simulink model "BalancingRobot"  (R2020a)
settings: Solver=FixedStepAuto  StartTime=0.0  StopTime=inf  FixedStep=.001  RelTol=1e-3  EnableMultiTasking=on
libraries: GPIO_Lib x9, REG_Lib x6, simulink x3, TIMERS_Lib x3, USART_Lib x1, STM32_Config_Lib x1
settings Model: Creator=brunj  LastModifiedBy=tuziz
settings DataIOCC: LimitDataPoints=on  SaveFormat=Array  ReturnWorkspaceOutputs=off
settings OptimizationCC: DefaultParameterBehavior=Inlined  PassReuseOutputArgsAs=Individual arguments  LifeSpan=1  EfficientTunableParamExpr=on
settings DebuggingCC: UnderspecifiedInitializationDetection=Classic  MergeDetectMultiDrivingBlocksExec=none  SolverPrmCheckMsg=warning  AllowSymbolicDim=off  StrictBusMsg=ErrorOnBusTreatedAsVector  SFUnexpectedBacktrackingDiag=warning  SFNoUnconditionalDefaultTransitionDiag=warning  SFUndirectedBroadcastEventsDiag=error  SFExecutionAtInitializationDiag=none  ArithmeticOperatorsInVariantConditions=warning
settings HardwareCC: ProdBitPerPointer=32  ProdBitPerSizeT=32  ProdBitPerPtrDiffT=32  ProdLargestAtomicInteger=Integer  ProdWordSize=32  ProdHWDeviceType=STMicroelectronics->STM32 32-bit Cortex-M
settings ModelReferenceCC: PropagateSignalLabelsOutOfModel=off
settings SFSimCC: SimUseLocalCustomCode=off  CompileTimeRecursionLimit=0  EnableRuntimeRecursion=off  MATLABDynamicMemAlloc=off  CustomCodeUndefinedFunction=UseInterfaceOnly
settings RTWCC: Description=stm32 (Embedded Target)  SystemTargetFile=stm32.tlc  TemplateMakefile=stm32.tmf  RTWUseLocalCustomCode=off  IncludeHyperlinkInReport=on
settings CodeAppCC: IgnoreCustomStorageClasses=off  CustomSymbolStrType=$N$R$M  SimulinkBlockComments=off
settings STFCustomTargetCC: ParMdlRefBuildCompliant=on  IncludeMdlTerminateFcn=off  CombineOutputUpdateFcns=on  ERTCustomFileBanners=on  SupportNonFinite=off  SupportComplex=off  SupportContinuousTime=off  SupportNonInlinedSFcns=off  RemoveResetFunc=on  ParenthesesLevel=Maximum  CastingMode=Standards  MATLABClassNameForMDSCustomization=Simulink.SoftwareTarget.ERTCustomization  SystemTargetFile=stm32.tlc
settings ERTTargetCC: MultiwordLength=2048  CompOptLevelCompliant=off  ConcurrentExecutionCompliant=off  IncludeMdlTerminateFcn=off  SupportNonFinite=off  SupportComplex=off  ParenthesesLevel=Maximum  CastingMode=Standards  ModelStepFunctionPrototypeControlCompliant=off  CPPClassGenCompliant=off  UseToolchainInfoCompliant=off  ExtModeTransport=1  ExtModeStaticAllocSize=256  ExtModeMexArgs=0,1,115200,10  InlinedParameterPlacement=NonHierarchical  ERTSrcFileBannerTemplate=sourceFileTemplate.cgt  ERTHdrFileBannerTemplate=sourceFileTemplate.cgt  ERTDataSrcFileTemplate=sourceFileTemplate.cgt  ERTDataHdrFileTemplate=sourceFileTemplate.cgt  ERTCustomFileTemplate=customRoutineProcess.tlc  ConvertIfToSwitch=off  SuppressUnreachableDefaultCases=off  EnableSignedLeftShifts=off  EnableSignedRightShifts=off
settings ConfigComp: CovMetricSettings=dw  CovHtmlReporting=on  CovSaveCumulativeToWorkspaceVar=on  CovSaveSingleToWorkspaceVar=on  CovExternalEMLEnable=off  CovSFcnEnable=off

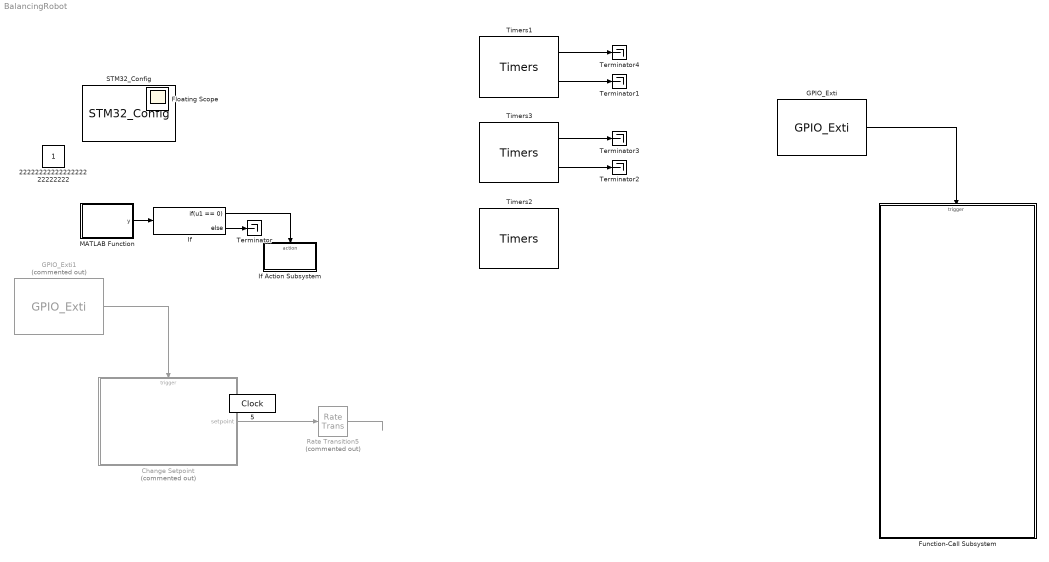
== system BalancingRobot ==
  Change Setpoint : Subsystem  Commented=on  TreatAsAtomicUnit=on
  Function-Call Subsystem : Subsystem  TreatAsAtomicUnit=on
  GPIO_Exti : GPIO_Lib/GPIO_Exti  Port_name=GPIOE  Pin_0=off  Pin_1=on  Pin_2=off  Pin_3=off  Pin_4=off  Pin_5=off  Pin_6=off  Pin_7=off  Pin_8=off  Pin_9=off  Pin_10=off  Pin_11=off  Pin_12=off  Pin_13=off  Pin_14=off  Pin_15=off  PinList=GPIOA0GPIOE1
      settings: SourceProductName=Target Support Package - STM32 Adapter
  GPIO_Exti1 : GPIO_Lib/GPIO_Exti  Commented=on  Port_name=GPIOA  Pin_0=on  Pin_1=off  Pin_2=off  Pin_3=off  Pin_4=off  Pin_5=off  Pin_6=off  Pin_7=off  Pin_8=off  Pin_9=off  Pin_10=off  Pin_11=off  Pin_12=off  Pin_13=off  Pin_14=off  Pin_15=off  PinList=GPIOA0GPIOE1
      settings: SourceProductName=Target Support Package - STM32 Adapter
  If : If  IfExpression=u1 == 0
  If Action Subsystem : Subsystem  TreatAsAtomicUnit=on
  MATLAB Function : MATLAB Function  TreatAsAtomicUnit=on
  Rate Transition5 : RateTransition  Commented=on  Deterministic=off
  STM32_Config : STM32_Config_Lib/STM32_Config  Priority=0  Project_Path=.\  Config_File=BalancingRobot.ioc  MCU_Name=STM32F407VGTx
      settings: SourceProductName=Target Support Package - STM32 Adapter
  Terminator{,1..4} (5 alike) : Terminator
  Timers1 : TIMERS_Lib/Timers  currentTIM=TIM3  TIM_Name=TIM3  sysUsingTimer=off  TIM_APBClock=84000000  TIM_Set_Clk=off  TIM_Prescaler=840-1  TIM_Clock=100000.00  Variable_frequency=off  TIM_Set_OutFreq=off  TIM_ARR=2000  Output_frequency=50.00  Repetition_counter=0  TIM_Mode=Up  TIM_DMA=none  TIM_IRQ=off  TIM_IRQ_ONLY=off  TIM_UP=off  TIM_TRG=off  TIM_COM=off  TIM_BRK=off  NbTIM=3  CH1_enable=on  CH1N_enable=off  CH1_type=Input_Capture  CH1_DMA=off  CH1_int=on  CH1_edge=Rising  CH1_div=1  CH1_variable_duty=off  CH1_set_pulse=off  CH1_output_duty=0.00  CH1_pulse=0  CH2_enable=off  CH2N_enable=off  CH2_type=Input_Capture  CH2_DMA=off  CH2_int=off  CH2_edge=Rising  CH2_div=1  CH2_variable_duty=off  CH2_set_pulse=off  CH2_output_duty=0.00  CH2_pulse=0  CH3_enable=off  CH3N_enable=off  CH3_type=Unknown  CH3_DMA=off  CH3_int=off  CH3_edge=Rising  CH3_div=1  CH3_variable_duty=off  CH3_set_pulse=off  CH3_output_duty=0.00  CH3_pulse=0  CH4_enable=off  CH4N_enable=off  CH4_type=Unknown  CH4_DMA=off  CH4_int=off  CH4_edge=Rising  CH4_div=1  CH4_variable_duty=off  CH4_set_pulse=off  CH4_output_duty=0.00  CH4_pulse=0
      settings: SourceProductName=Target Support Package - STM32 Adapter
  Timers2 : TIMERS_Lib/Timers  currentTIM=TIM9  TIM_Name=TIM9  sysUsingTimer=off  TIM_APBClock=168000000  TIM_Set_Clk=off  TIM_Prescaler=3359  TIM_Clock=50000.00  Variable_frequency=off  TIM_Set_OutFreq=off  TIM_ARR=100  Output_frequency=500.00  Repetition_counter=0  TIM_Mode=Up  TIM_DMA=none  TIM_IRQ=off  TIM_IRQ_ONLY=off  TIM_UP=off  TIM_TRG=off  TIM_COM=off  TIM_BRK=off  NbTIM=3  CH1_enable=on  CH1N_enable=off  CH1_type=Output_PWM  CH1_DMA=off  CH1_int=off  CH1_edge=Rising  CH1_div=1  CH1_variable_duty=off  CH1_set_pulse=off  CH1_output_duty=0.00  CH1_pulse=0  CH2_enable=on  CH2N_enable=off  CH2_type=Output_PWM  CH2_DMA=off  CH2_int=off  CH2_edge=Rising  CH2_div=1  CH2_variable_duty=off  CH2_set_pulse=off  CH2_output_duty=0.00  CH2_pulse=0  CH3_enable=off  CH3N_enable=off  CH3_type=Unknown  CH3_DMA=off  CH3_int=off  CH3_edge=Rising  CH3_div=1  CH3_variable_duty=off  CH3_set_pulse=off  CH3_output_duty=0.00  CH3_pulse=0  CH4_enable=off  CH4N_enable=off  CH4_type=Unknown  CH4_DMA=off  CH4_int=off  CH4_edge=Rising  CH4_div=1  CH4_variable_duty=off  CH4_set_pulse=off  CH4_output_duty=0.00  CH4_pulse=0
      settings: SourceProductName=Target Support Package - STM32 Adapter
  Timers3 : TIMERS_Lib/Timers  currentTIM=TIM2  TIM_Name=TIM2  sysUsingTimer=off  TIM_APBClock=84000000  TIM_Set_Clk=off  TIM_Prescaler=840-1  TIM_Clock=100000.00  Variable_frequency=off  TIM_Set_OutFreq=off  TIM_ARR=2000  Output_frequency=50.00  Repetition_counter=0  TIM_Mode=Up  TIM_DMA=none  TIM_IRQ=off  TIM_IRQ_ONLY=off  TIM_UP=off  TIM_TRG=off  TIM_COM=off  TIM_BRK=off  NbTIM=3  CH1_enable=on  CH1N_enable=off  CH1_type=Input_Capture  CH1_DMA=off  CH1_int=on  CH1_edge=Rising  CH1_div=1  CH1_variable_duty=off  CH1_set_pulse=off  CH1_output_duty=0.00  CH1_pulse=0  CH2_enable=off  CH2N_enable=off  CH2_type=Unknown  CH2_DMA=off  CH2_int=off  CH2_edge=Rising  CH2_div=1  CH2_variable_duty=off  CH2_set_pulse=off  CH2_output_duty=0.00  CH2_pulse=0  CH3_enable=off  CH3N_enable=off  CH3_type=Unknown  CH3_DMA=off  CH3_int=off  CH3_edge=Rising  CH3_div=1  CH3_variable_duty=off  CH3_set_pulse=off  CH3_output_duty=0.00  CH3_pulse=0  CH4_enable=off  CH4N_enable=off  CH4_type=Unknown  CH4_DMA=off  CH4_int=off  CH4_edge=Rising  CH4_div=1  CH4_variable_duty=off  CH4_set_pulse=off  CH4_output_duty=0.00  CH4_pulse=0
      settings: SourceProductName=Target Support Package - STM32 Adapter
  2222222222222222222222222 : Constant  IOType=siggen
  5 : DigitalClock  IOType=siggen
  Floating Scope : Scope
  wires:
  MATLAB Function/1(y) -> If/1
  If/1 -> If Action Subsystem/Action
  If/2 -> Terminator/1
  GPIO_Exti/1 -> Function-Call Subsystem/Trigger
  Rate Transition5/1 -> ?
  Change Setpoint/1(setpoint) -> Rate Transition5/1
  Timers1/1 -> Terminator4/1
  Timers3/2 -> Terminator2/1
  Timers3/1 -> Terminator3/1
  GPIO_Exti1/1 -> Change Setpoint/Trigger
  Timers1/2 -> Terminator1/1

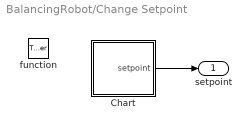
== system BalancingRobot/Change Setpoint ==
  function : TriggerPort  TriggerType=function-call  VariantControl=Variant  OutputDataType=int8
  Chart : Stateflow chart  TreatAsAtomicUnit=on
  setpoint : Outport
  wires:
  Chart/1(setpoint) -> setpoint/1

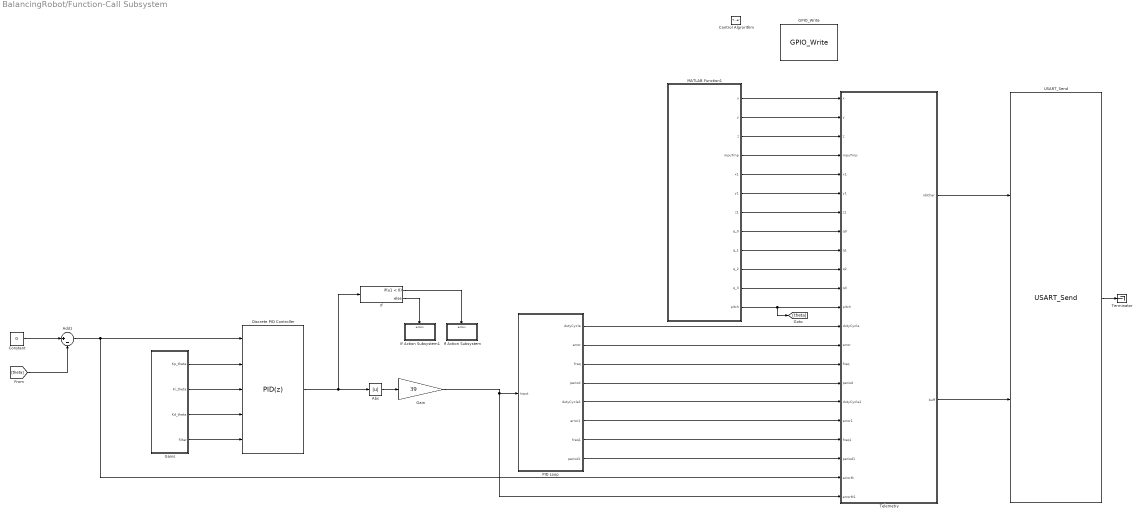
== system BalancingRobot/Function-Call Subsystem ==
  Control Algrorithm : TriggerPort  TriggerType=function-call  VariantControl=Variant
  Abs : Abs
  Add1 : Sum  Inputs=|+-  OutDataTypeStr=double
  Constant : Constant  Value=0
  Discrete PID Controller : simulink/Continuous/PID Controller  Controller=PID  Form=Parallel  TimeDomain=Discrete-time  UseExternalTs=off  SampleTime=-1  IntegratorMethod=Forward Euler  FilterMethod=Forward Euler  ControllerParametersSource=external  P=50.0  I=5  D=.5  UseFilter=on  N=100  TunerSelectOption=Transfer Function Based (PID Tuner App)  InitialConditionSource=internal  InitialConditionForIntegrator=0  InitialConditionForFilter=0  DifferentiatorICPrevScaledInput=0  ExternalReset=none  TrackingMode=off  Kt=1  LimitOutput=on  UpperSaturationLimit=39  LowerSaturationLimit=-39  LinearizeAsGain=off  AntiWindupMode=clamping  Kb=1  POutMin=[]  POutMax=[]  IOutMin=[]  IOutMax=[]  DOutMin=[]  DOutMax=[]  NOutMin=[]  NOutMax=[]  SumOutMin=[]  SumOutMax=[]  SaturationOutMin=[]  SaturationOutMax=[]  PParamMin=[]  PParamMax=[]  IParamMin=[]  IParamMax=[]  DParamMin=[]  DParamMax=[]  NParamMin=[]  NParamMax=[]  KbParamMin=[]  KbParamMax=[]  KtParamMin=[]  KtParamMax=[]  KbOutMin=[]  KbOutMax=[]  KtOutMin=[]  KtOutMax=[]  IntegratorOutMin=[]  IntegratorOutMax=[]  FilterOutMin=[]  FilterOutMax=[]  SumI1OutMin=[]  SumI1OutMax=[]  SumI2OutMin=[]  SumI2OutMax=[]  SumI3OutMin=[]  SumI3OutMax=[]  SumI4OutMin=[]  SumI4OutMax=[]  SumDOutMin=[]  SumDOutMax=[]  DifferentiatorOutMin=[]  DifferentiatorOutMax=[]  FilterDiffOutCoefMin=[]  FilterDiffOutCoefMax=[]  ReciprocalOutMin=[]  ReciprocalOutMax=[]  SumDenOutMin=[]  SumDenOutMax=[]  SumNumOutMin=[]  SumNumOutMax=[]  DivideOutMin=[]  DivideOutMax=[]  UdiffTsProdOutMin=[]  UdiffTsProdOutMax=[]  NTsProdOutMin=[]  NTsProdOutMax=[]  UintegralTsProdOutMin=[]  UintegralTsProdOutMax=[]  UngainTsProdOutMin=[]  UngainTsProdOutMax=[]  IntegratorContinuousStateAttributes=''  IntegratorStateMustResolveToSignalObject=off  IntegratorRTWStateStorageClass=Auto  FilterContinuousStateAttributes=''  FilterStateMustResolveToSignalObject=off  FilterRTWStateStorageClass=Auto  ParallelPVariant=ExternalParameters  IdealPVariant=Disabled  IVariant=ExternalParameters  DVariant=ExternalParameters  IntegratorVariant=Discrete  SatVariant=Enabled  AWVariant=DiscClampingParallel  PCopyVariant=Disabled  TRVariant=Disabled  FdbkBlocksVariant=Forward  IdealPFdbkVariant=Disabled  SatFdbkVariant=Disabled  DerivativeFilterVariant=ForwardEulerFilter  NVariant=ExternalParameters  NCopyVariant=Disabled  FilterICVariant=InternalICsFilter  IntegratorICVariant=InternalICs  ExternalResetVariant=Disabled  TRSumVariant=Passthrough  SumFdbkVariant=Disabled  SumVariant=Sum_PID  TsampFilterVariant=InternalTs  TsampNgainVariant=Passthrough  TsampIntegralVariant=Passthrough
  GPIO_Write : GPIO_Lib/GPIO_Write  Port_name=GPIOD  Pin0=off  Toggle_Pin0=off  Pin1=off  Toggle_Pin1=off  Pin2=off  Toggle_Pin2=off  Pin3=off  Toggle_Pin3=off  Pin4=off  Toggle_Pin4=off  Pin5=off  Toggle_Pin5=off  Pin6=off  Toggle_Pin6=off  Pin7=off  Toggle_Pin7=off  Pin8=off  Toggle_Pin8=off  Pin9=off  Toggle_Pin9=off  Pin10=off  Toggle_Pin10=off  Pin11=off  Toggle_Pin11=off  Pin12=off  Toggle_Pin12=off  Pin13=off  Toggle_Pin13=off  Pin14=off  Toggle_Pin14=off  Pin15=on  Toggle_Pin15=on  PinList="GPIOD1   2   3   4  12  13  14  15"
      settings: SourceProductName=Target Support Package - STM32 Adapter
  Gain : Gain  Gain=39
  Gains : MATLAB Function  TreatAsAtomicUnit=on
  If : If  IfExpression=u1 < 0
  If Action Subsystem : Subsystem  TreatAsAtomicUnit=on
  If Action Subsystem1 : Subsystem  TreatAsAtomicUnit=on
  MATLAB Function1 : MATLAB Function  Priority=0  TreatAsAtomicUnit=on
  PID Loop : Subsystem  TreatAsAtomicUnit=on
  Telemetry : MATLAB Function  TreatAsAtomicUnit=on
  Terminator : Terminator
  USART_Send : USART_Lib/USART_Send  USART_name=USART3  Buff_size=199  nbUsart=1  usartMode=Asynchronous  usartDma_Rx=off  usartDma_Tx=off  usartIt=on
      settings: SourceProductName=Target Support Package - STM32 Adapter
  wires:
  Telemetry/2(buff) -> USART_Send/2
  Telemetry/1(nbChar) -> USART_Send/1
  USART_Send/1 -> Terminator/1
  MATLAB Function1/3(z) -> Telemetry/3(z)
  MATLAB Function1/1(x) -> Telemetry/1(x)
  MATLAB Function1/2(y) -> Telemetry/2(y)
  MATLAB Function1/4(mpuTmp) -> Telemetry/4(mpuTmp)
  MATLAB Function1/5(x1) -> Telemetry/5(x1)
  MATLAB Function1/6(y1) -> Telemetry/6(y1)
  MATLAB Function1/7(z1) -> Telemetry/7(z1)
  MATLAB Function1/8(q_0) -> Telemetry/8(q0)
  MATLAB Function1/9(q_1) -> Telemetry/9(q1)
  MATLAB Function1/10(q_2) -> Telemetry/10(q2)
  MATLAB Function1/11(q_3) -> Telemetry/11(q3)
  MATLAB Function1/12(pitch) -> [theta], Telemetry/12(pitch)
  PID Loop/1(dutyCycle) -> Telemetry/13(dutyCycle)
  PID Loop/2(error) -> Telemetry/14(error)
  PID Loop/3(freq) -> Telemetry/15(freq)
  PID Loop/4(period) -> Telemetry/16(period)
  PID Loop/5(dutyCycle1) -> Telemetry/17(dutyCycle1)
  PID Loop/6(error1) -> Telemetry/18(error1)
  PID Loop/7(freq1) -> Telemetry/19(freq1)
  PID Loop/8(period1) -> Telemetry/20(period1)
  If/1 -> If Action Subsystem/Action
  If/2 -> If Action Subsystem1/Action
  Discrete PID Controller/1 -> If/1, Abs/1
  Add1/1 -> Discrete PID Controller/1, Telemetry/21(errorM)
  Gains/1(Kp_theta) -> Discrete PID Controller/2
  Gains/2(Ki_theta) -> Discrete PID Controller/3
  Gains/3(Kd_theta) -> Discrete PID Controller/4
  Gains/4(filter) -> Discrete PID Controller/5
  Gain/1 -> Telemetry/22(errorM1), PID Loop/1(Input)
  Constant/1 -> Add1/1
  Abs/1 -> Gain/1
  [theta] -> Add1/2

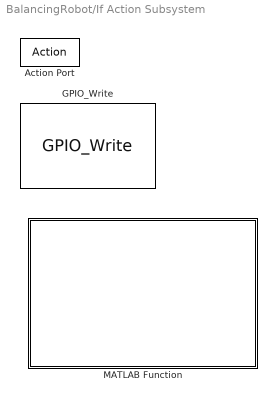
== system BalancingRobot/If Action Subsystem ==
  Action Port : ActionPort  ActionPortLabel=if(u1 == 0)
  GPIO_Write : GPIO_Lib/GPIO_Write  Port_name=GPIOD  Pin0=off  Toggle_Pin0=off  Pin1=off  Toggle_Pin1=off  Pin2=off  Toggle_Pin2=off  Pin3=off  Toggle_Pin3=off  Pin4=off  Toggle_Pin4=off  Pin5=off  Toggle_Pin5=off  Pin6=off  Toggle_Pin6=off  Pin7=off  Toggle_Pin7=off  Pin8=off  Toggle_Pin8=off  Pin9=off  Toggle_Pin9=off  Pin10=off  Toggle_Pin10=off  Pin11=off  Toggle_Pin11=off  Pin12=on  Toggle_Pin12=on  Pin13=off  Toggle_Pin13=off  Pin14=off  Toggle_Pin14=off  Pin15=off  Toggle_Pin15=off  PinList="GPIOD1   2   3   4  12  13  14  15"
      settings: SourceProductName=Target Support Package - STM32 Adapter
  MATLAB Function : MATLAB Function  TreatAsAtomicUnit=on

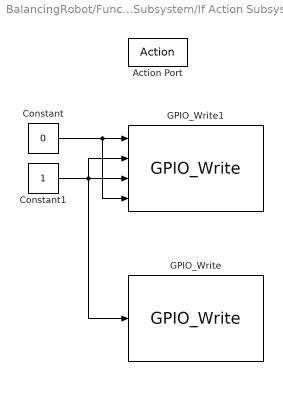
== system BalancingRobot/Function-Call Subsystem/If Action Subsystem ==
  Action Port : ActionPort  ActionPortLabel=if(u1 < 0)
  Constant : Constant  Value=0
  Constant1 : Constant
  GPIO_Write : GPIO_Lib/GPIO_Write  Port_name=GPIOD  Pin0=off  Toggle_Pin0=off  Pin1=off  Toggle_Pin1=off  Pin2=off  Toggle_Pin2=off  Pin3=off  Toggle_Pin3=off  Pin4=off  Toggle_Pin4=off  Pin5=off  Toggle_Pin5=off  Pin6=off  Toggle_Pin6=off  Pin7=off  Toggle_Pin7=off  Pin8=off  Toggle_Pin8=off  Pin9=off  Toggle_Pin9=off  Pin10=off  Toggle_Pin10=off  Pin11=off  Toggle_Pin11=off  Pin12=off  Toggle_Pin12=off  Pin13=on  Toggle_Pin13=off  Pin14=off  Toggle_Pin14=off  Pin15=off  Toggle_Pin15=off  PinList="GPIOD1   2   3   4  12  13  14  15"
      settings: SourceProductName=Target Support Package - STM32 Adapter
  GPIO_Write1 : GPIO_Lib/GPIO_Write  Port_name=GPIOD  Pin0=off  Toggle_Pin0=off  Pin1=on  Toggle_Pin1=off  Pin2=on  Toggle_Pin2=off  Pin3=on  Toggle_Pin3=off  Pin4=on  Toggle_Pin4=off  Pin5=off  Toggle_Pin5=off  Pin6=off  Toggle_Pin6=off  Pin7=off  Toggle_Pin7=off  Pin8=off  Toggle_Pin8=off  Pin9=off  Toggle_Pin9=off  Pin10=off  Toggle_Pin10=off  Pin11=off  Toggle_Pin11=off  Pin12=off  Toggle_Pin12=off  Pin13=off  Toggle_Pin13=off  Pin14=off  Toggle_Pin14=off  Pin15=off  Toggle_Pin15=off  PinList="GPIOD1   2   3   4  12  13  14  15"
      settings: SourceProductName=Target Support Package - STM32 Adapter
  wires:
  Constant/1 -> GPIO_Write1/4, GPIO_Write1/1
  Constant1/1 -> GPIO_Write/1, GPIO_Write1/3, GPIO_Write1/2

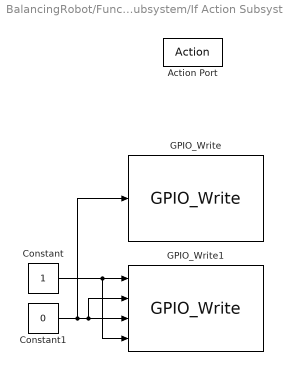
== system BalancingRobot/Function-Call Subsystem/If Action Subsystem1 ==
  Action Port : ActionPort  ActionPortLabel=else
  Constant : Constant
  Constant1 : Constant  Value=0
  GPIO_Write : GPIO_Lib/GPIO_Write  Port_name=GPIOD  Pin0=off  Toggle_Pin0=off  Pin1=off  Toggle_Pin1=off  Pin2=off  Toggle_Pin2=off  Pin3=off  Toggle_Pin3=off  Pin4=off  Toggle_Pin4=off  Pin5=off  Toggle_Pin5=off  Pin6=off  Toggle_Pin6=off  Pin7=off  Toggle_Pin7=off  Pin8=off  Toggle_Pin8=off  Pin9=off  Toggle_Pin9=off  Pin10=off  Toggle_Pin10=off  Pin11=off  Toggle_Pin11=off  Pin12=off  Toggle_Pin12=off  Pin13=on  Toggle_Pin13=off  Pin14=off  Toggle_Pin14=off  Pin15=off  Toggle_Pin15=off  PinList="GPIOD1   2   3   4  12  13  14  15"
      settings: SourceProductName=Target Support Package - STM32 Adapter
  GPIO_Write1 : GPIO_Lib/GPIO_Write  Port_name=GPIOD  Pin0=off  Toggle_Pin0=off  Pin1=on  Toggle_Pin1=off  Pin2=on  Toggle_Pin2=off  Pin3=on  Toggle_Pin3=off  Pin4=on  Toggle_Pin4=off  Pin5=off  Toggle_Pin5=off  Pin6=off  Toggle_Pin6=off  Pin7=off  Toggle_Pin7=off  Pin8=off  Toggle_Pin8=off  Pin9=off  Toggle_Pin9=off  Pin10=off  Toggle_Pin10=off  Pin11=off  Toggle_Pin11=off  Pin12=off  Toggle_Pin12=off  Pin13=off  Toggle_Pin13=off  Pin14=off  Toggle_Pin14=off  Pin15=off  Toggle_Pin15=off  PinList="GPIOD1   2   3   4  12  13  14  15"
      settings: SourceProductName=Target Support Package - STM32 Adapter
  wires:
  Constant/1 -> GPIO_Write1/4, GPIO_Write1/1
  Constant1/1 -> GPIO_Write/1, GPIO_Write1/3, GPIO_Write1/2

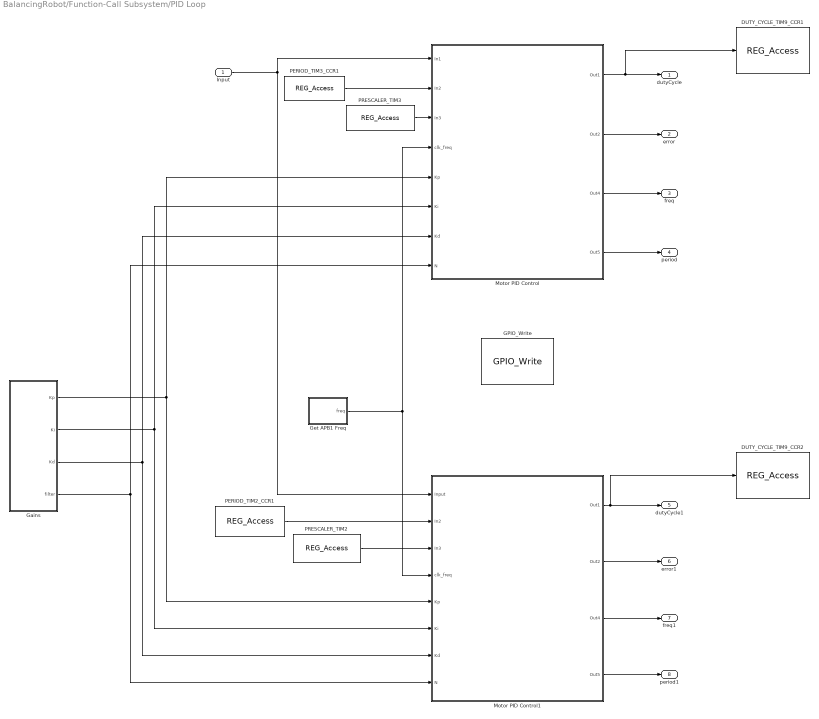
== system BalancingRobot/Function-Call Subsystem/PID Loop ==
  Input : Inport
  DUTY_CYCLE_TIM9_CCR1 : REG_Lib/REG_Access  Peripheral=TIM9  RegName=CCR1  RegRead=off  RegWrite=on  RegValueIn=on  RegEqual=on  RegAnd=off  RegOr=off  RegComplement=off  currentPeriph=I2C1
      settings: SourceProductName=Target Support Package - STM32 Adapter
  DUTY_CYCLE_TIM9_CCR2 : REG_Lib/REG_Access  Peripheral=TIM9  RegName=CCR2  RegRead=off  RegWrite=on  RegValueIn=on  RegEqual=on  RegAnd=off  RegOr=off  RegComplement=off  currentPeriph=TIM9
      settings: SourceProductName=Target Support Package - STM32 Adapter
  GPIO_Write : GPIO_Lib/GPIO_Write  Port_name=GPIOD  Pin0=off  Toggle_Pin0=off  Pin1=off  Toggle_Pin1=off  Pin2=off  Toggle_Pin2=off  Pin3=off  Toggle_Pin3=off  Pin4=off  Toggle_Pin4=off  Pin5=off  Toggle_Pin5=off  Pin6=off  Toggle_Pin6=off  Pin7=off  Toggle_Pin7=off  Pin8=off  Toggle_Pin8=off  Pin9=off  Toggle_Pin9=off  Pin10=off  Toggle_Pin10=off  Pin11=off  Toggle_Pin11=off  Pin12=off  Toggle_Pin12=off  Pin13=off  Toggle_Pin13=off  Pin14=on  Toggle_Pin14=on  Pin15=off  Toggle_Pin15=off  PinList="GPIOD1   2   3   4  12  13  14  15"
      settings: SourceProductName=Target Support Package - STM32 Adapter
  Gains : MATLAB Function  TreatAsAtomicUnit=on
  Get APB1 Freq : MATLAB Function  TreatAsAtomicUnit=on
  Motor PID Control : Subsystem
  Motor PID Control1 : Subsystem
  PERIOD_TIM2_CCR1 : REG_Lib/REG_Access  Peripheral=TIM2  RegName=CCR1  RegRead=on  RegWrite=off  RegValueIn=off  RegEqual=on  RegAnd=off  RegOr=off  RegComplement=off  currentPeriph=I2C1
      settings: SourceProductName=Target Support Package - STM32 Adapter
  PERIOD_TIM3_CCR1 : REG_Lib/REG_Access  Peripheral=TIM3  RegName=CCR1  RegRead=on  RegWrite=off  RegValueIn=off  RegEqual=on  RegAnd=off  RegOr=off  RegComplement=off  currentPeriph=I2C1
      settings: SourceProductName=Target Support Package - STM32 Adapter
  PRESCALER_TIM2 : REG_Lib/REG_Access  Peripheral=TIM2  RegName=PSC  RegRead=on  RegWrite=off  RegValueIn=off  RegEqual=on  RegAnd=off  RegOr=off  RegComplement=off  currentPeriph=I2C1
      settings: SourceProductName=Target Support Package - STM32 Adapter
  PRESCALER_TIM3 : REG_Lib/REG_Access  Peripheral=TIM3  RegName=PSC  RegRead=on  RegWrite=off  RegValueIn=off  RegEqual=on  RegAnd=off  RegOr=off  RegComplement=off  currentPeriph=I2C1
      settings: SourceProductName=Target Support Package - STM32 Adapter
  dutyCycle : Outport
  error : Outport  Port=2
  freq : Outport  Port=3
  period : Outport  Port=4
  dutyCycle1 : Outport  Port=5
  error1 : Outport  Port=6
  freq1 : Outport  Port=7
  period1 : Outport  Port=8
  wires:
  Motor PID Control/1(Out1) -> DUTY_CYCLE_TIM9_CCR1/1, dutyCycle/1
  PERIOD_TIM3_CCR1/1 -> Motor PID Control/2(In2)
  Motor PID Control/2(Out2) -> error/1
  Motor PID Control/3(Out4) -> freq/1
  Motor PID Control/4(Out5) -> period/1
  Input/1 -> Motor PID Control1/1(Input), Motor PID Control/1(In1)
  Motor PID Control1/4(Out5) -> period1/1
  Motor PID Control1/3(Out4) -> freq1/1
  Motor PID Control1/2(Out2) -> error1/1
  PERIOD_TIM2_CCR1/1 -> Motor PID Control1/2(In2)
  Motor PID Control1/1(Out1) -> DUTY_CYCLE_TIM9_CCR2/1, dutyCycle1/1
  Get APB1 Freq/1(freq) -> Motor PID Control/4(clk_freq), Motor PID Control1/4(clk_freq)
  PRESCALER_TIM3/1 -> Motor PID Control/3(In3)
  PRESCALER_TIM2/1 -> Motor PID Control1/3(In3)
  Gains/1(Kp) -> Motor PID Control/5(Kp), Motor PID Control1/5(Kp)
  Gains/2(Ki) -> Motor PID Control/6(Ki), Motor PID Control1/6(Ki)
  Gains/3(Kd) -> Motor PID Control/7(Kd), Motor PID Control1/7(Kd)
  Gains/4(filter) -> Motor PID Control/8(N), Motor PID Control1/8(N)

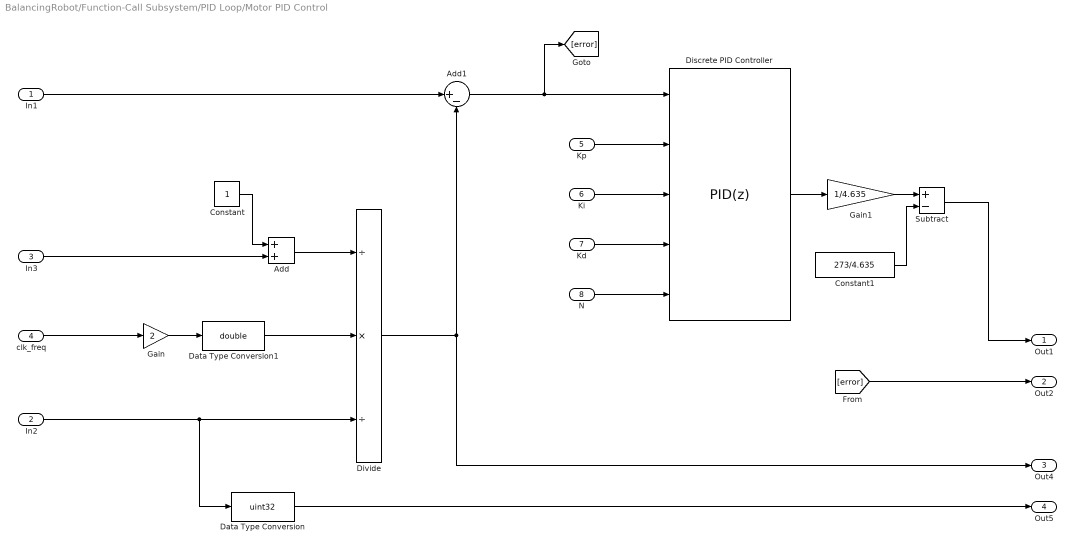
== system BalancingRobot/Function-Call Subsystem/PID Loop/Motor PID Control ==
  In1 : Inport
  In2 : Inport  Port=2
  In3 : Inport  Port=3
  clk_freq : Inport  Port=4
  Kp : Inport  Port=5
  Ki : Inport  Port=6
  Kd : Inport  Port=7
  N : Inport  Port=8
  Add : Sum  OutDataTypeStr=double
  Add1 : Sum  Inputs=|+-  OutDataTypeStr=double
  Constant : Constant  OutDataTypeStr=double
  Constant1 : Constant  Value=273/4.635
  Data Type Conversion : DataTypeConversion  OutDataTypeStr=uint32
  Data Type Conversion1 : DataTypeConversion  OutDataTypeStr=double
  Discrete PID Controller : simulink/Continuous/PID Controller  Controller=PID  Form=Parallel  TimeDomain=Discrete-time  UseExternalTs=off  SampleTime=-1  IntegratorMethod=Forward Euler  FilterMethod=Forward Euler  ControllerParametersSource=external  P=50.0  I=5  D=.5  UseFilter=on  N=100  TunerSelectOption=Transfer Function Based (PID Tuner App)  InitialConditionSource=internal  InitialConditionForIntegrator=0  InitialConditionForFilter=0  DifferentiatorICPrevScaledInput=0  ExternalReset=none  TrackingMode=off  Kt=1  LimitOutput=on  UpperSaturationLimit=700  LowerSaturationLimit=0  LinearizeAsGain=off  AntiWindupMode=clamping  Kb=1  POutMin=[]  POutMax=[]  IOutMin=[]  IOutMax=[]  DOutMin=[]  DOutMax=[]  NOutMin=[]  NOutMax=[]  SumOutMin=[]  SumOutMax=[]  SaturationOutMin=[]  SaturationOutMax=[]  PParamMin=[]  PParamMax=[]  IParamMin=[]  IParamMax=[]  DParamMin=[]  DParamMax=[]  NParamMin=[]  NParamMax=[]  KbParamMin=[]  KbParamMax=[]  KtParamMin=[]  KtParamMax=[]  KbOutMin=[]  KbOutMax=[]  KtOutMin=[]  KtOutMax=[]  IntegratorOutMin=[]  IntegratorOutMax=[]  FilterOutMin=[]  FilterOutMax=[]  SumI1OutMin=[]  SumI1OutMax=[]  SumI2OutMin=[]  SumI2OutMax=[]  SumI3OutMin=[]  SumI3OutMax=[]  SumI4OutMin=[]  SumI4OutMax=[]  SumDOutMin=[]  SumDOutMax=[]  DifferentiatorOutMin=[]  DifferentiatorOutMax=[]  FilterDiffOutCoefMin=[]  FilterDiffOutCoefMax=[]  ReciprocalOutMin=[]  ReciprocalOutMax=[]  SumDenOutMin=[]  SumDenOutMax=[]  SumNumOutMin=[]  SumNumOutMax=[]  DivideOutMin=[]  DivideOutMax=[]  UdiffTsProdOutMin=[]  UdiffTsProdOutMax=[]  NTsProdOutMin=[]  NTsProdOutMax=[]  UintegralTsProdOutMin=[]  UintegralTsProdOutMax=[]  UngainTsProdOutMin=[]  UngainTsProdOutMax=[]  IntegratorContinuousStateAttributes=''  IntegratorStateMustResolveToSignalObject=off  IntegratorRTWStateStorageClass=Auto  FilterContinuousStateAttributes=''  FilterStateMustResolveToSignalObject=off  FilterRTWStateStorageClass=Auto  ParallelPVariant=ExternalParameters  IdealPVariant=Disabled  IVariant=ExternalParameters  DVariant=ExternalParameters  IntegratorVariant=Discrete  SatVariant=Enabled  AWVariant=DiscClampingParallel  PCopyVariant=Disabled  TRVariant=Disabled  FdbkBlocksVariant=Forward  IdealPFdbkVariant=Disabled  SatFdbkVariant=Disabled  DerivativeFilterVariant=ForwardEulerFilter  NVariant=ExternalParameters  NCopyVariant=Disabled  FilterICVariant=InternalICsFilter  IntegratorICVariant=InternalICs  ExternalResetVariant=Disabled  TRSumVariant=Passthrough  SumFdbkVariant=Disabled  SumVariant=Sum_PID  TsampFilterVariant=InternalTs  TsampNgainVariant=Passthrough  TsampIntegralVariant=Passthrough
  Divide : Product  Inputs=/*/  OutDataTypeStr=double
  Gain : Gain  Gain=2  ParamDataTypeStr=double  OutDataTypeStr=double
  Gain1 : Gain  Gain=1/4.635  OutDataTypeStr=double
  Subtract : Sum  Inputs=+-
  Out1 : Outport
  Out2 : Outport  Port=2
  Out4 : Outport  Port=3
  Out5 : Outport  Port=4
  wires:
  In3/1 -> Add/2
  Data Type Conversion/1 -> Out5/1
  Add1/1 -> [error], Discrete PID Controller/1
  Constant/1 -> Add/1
  In2/1 -> Data Type Conversion/1, Divide/3
  Add/1 -> Divide/1
  Divide/1 -> Out4/1, Add1/2
  Discrete PID Controller/1 -> Gain1/1
  Kd/1 -> Discrete PID Controller/4
  clk_freq/1 -> Gain/1
  Kp/1 -> Discrete PID Controller/2
  Gain/1 -> Data Type Conversion1/1
  Ki/1 -> Discrete PID Controller/3
  [error] -> Out2/1
  Data Type Conversion1/1 -> Divide/2
  N/1 -> Discrete PID Controller/5
  In1/1 -> Add1/1
  Gain1/1 -> Subtract/1
  Subtract/1 -> Out1/1
  Constant1/1 -> Subtract/2

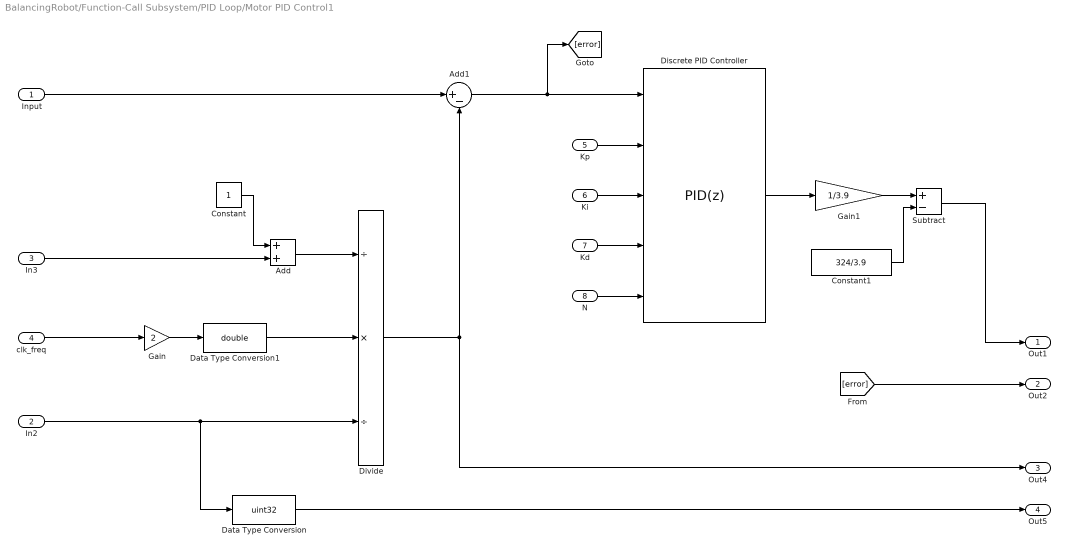
== system BalancingRobot/Function-Call Subsystem/PID Loop/Motor PID Control1 ==
  Input : Inport
  In2 : Inport  Port=2
  In3 : Inport  Port=3
  clk_freq : Inport  Port=4
  Kp : Inport  Port=5
  Ki : Inport  Port=6
  Kd : Inport  Port=7
  N : Inport  Port=8
  Add : Sum  OutDataTypeStr=double
  Add1 : Sum  Inputs=|+-  OutDataTypeStr=double
  Constant : Constant  OutDataTypeStr=double
  Constant1 : Constant  Value=324/3.9
  Data Type Conversion : DataTypeConversion  OutDataTypeStr=uint32
  Data Type Conversion1 : DataTypeConversion  OutDataTypeStr=double
  Discrete PID Controller : simulink/Continuous/PID Controller  Controller=PID  Form=Parallel  TimeDomain=Discrete-time  UseExternalTs=off  SampleTime=-1  IntegratorMethod=Forward Euler  FilterMethod=Forward Euler  ControllerParametersSource=external  P=50.0  I=5  D=.5  UseFilter=on  N=100  TunerSelectOption=Transfer Function Based (PID Tuner App)  InitialConditionSource=internal  InitialConditionForIntegrator=0  InitialConditionForFilter=0  DifferentiatorICPrevScaledInput=0  ExternalReset=none  TrackingMode=off  Kt=1  LimitOutput=on  UpperSaturationLimit=700  LowerSaturationLimit=0  LinearizeAsGain=off  AntiWindupMode=clamping  Kb=1  POutMin=[]  POutMax=[]  IOutMin=[]  IOutMax=[]  DOutMin=[]  DOutMax=[]  NOutMin=[]  NOutMax=[]  SumOutMin=[]  SumOutMax=[]  SaturationOutMin=[]  SaturationOutMax=[]  PParamMin=[]  PParamMax=[]  IParamMin=[]  IParamMax=[]  DParamMin=[]  DParamMax=[]  NParamMin=[]  NParamMax=[]  KbParamMin=[]  KbParamMax=[]  KtParamMin=[]  KtParamMax=[]  KbOutMin=[]  KbOutMax=[]  KtOutMin=[]  KtOutMax=[]  IntegratorOutMin=[]  IntegratorOutMax=[]  FilterOutMin=[]  FilterOutMax=[]  SumI1OutMin=[]  SumI1OutMax=[]  SumI2OutMin=[]  SumI2OutMax=[]  SumI3OutMin=[]  SumI3OutMax=[]  SumI4OutMin=[]  SumI4OutMax=[]  SumDOutMin=[]  SumDOutMax=[]  DifferentiatorOutMin=[]  DifferentiatorOutMax=[]  FilterDiffOutCoefMin=[]  FilterDiffOutCoefMax=[]  ReciprocalOutMin=[]  ReciprocalOutMax=[]  SumDenOutMin=[]  SumDenOutMax=[]  SumNumOutMin=[]  SumNumOutMax=[]  DivideOutMin=[]  DivideOutMax=[]  UdiffTsProdOutMin=[]  UdiffTsProdOutMax=[]  NTsProdOutMin=[]  NTsProdOutMax=[]  UintegralTsProdOutMin=[]  UintegralTsProdOutMax=[]  UngainTsProdOutMin=[]  UngainTsProdOutMax=[]  IntegratorContinuousStateAttributes=''  IntegratorStateMustResolveToSignalObject=off  IntegratorRTWStateStorageClass=Auto  FilterContinuousStateAttributes=''  FilterStateMustResolveToSignalObject=off  FilterRTWStateStorageClass=Auto  ParallelPVariant=ExternalParameters  IdealPVariant=Disabled  IVariant=ExternalParameters  DVariant=ExternalParameters  IntegratorVariant=Discrete  SatVariant=Enabled  AWVariant=DiscClampingParallel  PCopyVariant=Disabled  TRVariant=Disabled  FdbkBlocksVariant=Forward  IdealPFdbkVariant=Disabled  SatFdbkVariant=Disabled  DerivativeFilterVariant=ForwardEulerFilter  NVariant=ExternalParameters  NCopyVariant=Disabled  FilterICVariant=InternalICsFilter  IntegratorICVariant=InternalICs  ExternalResetVariant=Disabled  TRSumVariant=Passthrough  SumFdbkVariant=Disabled  SumVariant=Sum_PID  TsampFilterVariant=InternalTs  TsampNgainVariant=Passthrough  TsampIntegralVariant=Passthrough
  Divide : Product  Inputs=/*/  OutDataTypeStr=double
  Gain : Gain  Gain=2  ParamDataTypeStr=double  OutDataTypeStr=double
  Gain1 : Gain  Gain=1/3.9  OutDataTypeStr=double
  Subtract : Sum  Inputs=+-
  Out1 : Outport
  Out2 : Outport  Port=2
  Out4 : Outport  Port=3
  Out5 : Outport  Port=4
  wires:
  Input/1 -> Add1/1
  N/1 -> Discrete PID Controller/5
  Data Type Conversion1/1 -> Divide/2
  [error] -> Out2/1
  Ki/1 -> Discrete PID Controller/3
  Gain/1 -> Data Type Conversion1/1
  Kp/1 -> Discrete PID Controller/2
  clk_freq/1 -> Gain/1
  Kd/1 -> Discrete PID Controller/4
  Discrete PID Controller/1 -> Gain1/1
  Divide/1 -> Add1/2, Out4/1
  Add/1 -> Divide/1
  In2/1 -> Divide/3, Data Type Conversion/1
  Constant/1 -> Add/1
  Add1/1 -> Discrete PID Controller/1, [error]
  Data Type Conversion/1 -> Out5/1
  In3/1 -> Add/2
  Subtract/1 -> Out1/1
  Constant1/1 -> Subtract/2
  Gain1/1 -> Subtract/1

== matlab function BalancingRobot/Function-Call Subsystem/PID Loop/Gains ==
  data: Kp output; Ki output; Kd output; filter output
function [Kp,Ki,Kd,filter] = fcn()
if coder.target('Sfun')
    % Executing in MATLAB, Buff is null
    Kp = double(0);
    Ki = double(0);
    Kd = double(0);
    filter  = double(0);
else
    coder.cinclude('pid_gains.h');

    % Executing in the generated code.
    Kp = coder.ceval('getKp');
    Ki = coder.ceval('getKi');
    Kd = coder.ceval('getKd');
    filter  = coder.ceval('getN');
end
end

== matlab function BalancingRobot/Function-Call Subsystem/PID Loop/Get APB1 Freq ==
  data: freq output
function freq = fcn()
if coder.target('Sfun')
    % Executing in MATLAB, Buff is null
    freq = double(0);
else
    coder.cinclude('stm32f4xx_hal_rcc.h');
    
    % Executing in the generated code.
    freq = coder.ceval('HAL_RCC_GetPCLK1Freq');
end
end

== matlab function BalancingRobot/Function-Call Subsystem/Gains ==
  data: Kp_theta output; Ki_theta output; Kd_theta output; filter output
function [Kp_theta,Ki_theta,Kd_theta,filter] = fcn()
if coder.target('Sfun')
    % Executing in MATLAB, Buff is null
    Kp_theta = double(0);
    Ki_theta = double(0);
    Kd_theta = double(0);
    filter  = double(0);
else
    coder.cinclude('pid_gains.h');

    % Executing in the generated code.
    Kp_theta = coder.ceval('getKp_theta');
    Ki_theta = coder.ceval('getKi_theta');
    Kd_theta = coder.ceval('getKd_theta');
    filter  = coder.ceval('getN');
end
end

== matlab function BalancingRobot/MATLAB Function ==
  data: y output
function y = fcn()
if coder.target('Sfun')
    % Executing in MATLAB, Buff is null
    y = int8(0);
else
    coder.cinclude('mpu6050.h');

    % Executing in the generated code.
    y = coder.ceval('isSetup');
    
end
end

== matlab function BalancingRobot/Function-Call Subsystem/Telemetry ==
  data: x input; nbChar output uint16 size=1; buff output uint32 size=1; y input; z input; mpuTmp input; x1 input; y1 input; z1 input; q0 input; q1 input; q2 input; q3 input; pitch input; dutyCycle input; error input; freq input; period input; dutyCycle1 input; error1 input; freq1 input; period1 input; errorM input; errorM1 input
function [nbChar, buff] = convert(x,y,z,mpuTmp,x1,y1,z1,q0,q1,q2,q3,pitch,dutyCycle,error,freq,period,dutyCycle1,error1,freq1,period1,errorM,errorM1)
if coder.target('Sfun')
    % Executing in MATLAB, Buff is null
    buff = uint32(0);
    nbChar = uint16(0);
else
    coder.cinclude('stdio.h');
    coder.cinclude('main.h');
    coder.cinclude('getBuffPtr.h');
    coder.cinclude('string.h');

    % Executing in the generated code.
    string = char(zeros(1,205));
    stringSize = uint16(size(string,2));
    stringFormat = char(['%7.3f,','%7.3f,','%7.3f,','%7.3f,','%7.3f,','%7.3f,','%7.3f,','%7.3f,','%7.3f,','%7.3f,','%7.3f,','%7.3f,','%7u,','%9.2f,','%9.2f,','%9.2f,','%9.2f,','%9u,','%11.2f,','%9.2f,','%11.2f,','%9.2f',13,10,0]);
    coder.ceval('snprintf',coder.wref(string),stringSize,coder.rref(stringFormat),x,y,z,mpuTmp,x1,y1,z1,q0,q1,q2,q3,pitch,period,error,errorM,freq,dutyCycle,period1,error1,errorM1,freq1,dutyCycle1);
    buff = coder.ceval('getBuffPtr',coder.rref(string));
    nbChar = coder.ceval('strlen',string);
end
end

== stateflow chart BalancingRobot/Change Setpoint/Chart ==
  state S1
    setpoint=150.00;
  state S2
    setpoint=300.00;
  state S4
    setpoint=600.00;
  state S3
    setpoint=450.00;
  (default) -> S1
  S1 -> S2
  S4 -> S1
  S2 -> S3
  S3 -> S4
  data: setpoint output

== matlab function BalancingRobot/If Action Subsystem/MATLAB Function ==
function fcn()
if coder.target('Sfun')
    % Executing in MATLAB, Buff is null
else
    coder.cinclude('mpu6050.h');

    % Executing in the generated code.
    coder.ceval('setFlag');
    coder.ceval('setupMPU6050');
    
end
end

== matlab function BalancingRobot/Function-Call Subsystem/MATLAB Function1 ==
  data: x output; y output; z output; mpuTmp output; x1 output; y1 output; z1 output; q_0 output; q_1 output; q_2 output; q_3 output; pitch output
function [x,y,z,mpuTmp,x1,y1,z1,q_0,q_1,q_2,q_3,pitch]= read_mpu()
if coder.target('Sfun')
    % Executing in MATLAB, Buff is null
    x = double(0);
    y = double(0);
    z = double(0);
    mpuTmp = double(0);
    x1 = double(0);
    y1 = double(0);
    z1 = double(0);
    q_0 = double(0);    
    q_1 = double(0);
    q_2 = double(0);
    q_3 = double(0);
    pitch = double(0);
else
    coder.cinclude('mpu6050.h');
    coder.cinclude('MadgwickAHRS.h');
    
    % Executing in the generated code.
    coder.ceval('mpu6050_read_sensors');
    
    x = coder.ceval('Accel_x_g');    
    y = coder.ceval('Accel_y_g'); 
    z = coder.ceval('Accel_z_g');
    
    mpuTmp = coder.ceval('Mpu_temp_c');
    
    x1 = coder.ceval('Gyro_x_rad');    
    y1 = coder.ceval('Gyro_y_rad'); 
    z1 = coder.ceval('Gyro_z_rad'); 
    
    q_0 = coder.ceval('getQ_0');    
    q_1 = coder.ceval('getQ_1');
    q_2 = coder.ceval('getQ_2');
    q_3 = coder.ceval('getQ_3');
    pitch = coder.ceval('getPitch');
    
    coder.ceval('MadgwickAHRSupdateIMU', x1, y1, z1, x, y, z);
end
